simulink model "WTPG_SIM"  (R2022a)
settings: Solver=FixedStepDiscrete  StartTime=0.0  StopTime=1.08  FixedStep=0.04  RelTol=1e-3
PreLoadFcn:
  | listing = dir;
  | if (contains([listing .name], 'TCAF')) && (contains([listing .name], 'MAP'))
  |     addpath('./TCAF', './MAP');
  |     addpath( genpath('./MAP') );
  | elseif (contains([listing .name], 'WTPG.slx'))
  |     addpath('../TCAF', '../MAP');
  |     addpath( genpath('../MAP') );
  | else
  | 
  | end
  | 
  | load('BusStructureWTPG.mat');
  | load('TRN\BusStructureTRN.mat');
InitFcn:
  | listing = dir;
  | if (contains([listing .name], 'TCAF')) && (contains([listing .name], 'MAP'))
  |     addpath('./TCAF', './MAP');
  |     addpath( genpath('./MAP') );
  | elseif (contains([listing .name], 'WTPG.slx'))
  |     addpath('../TCAF', '../MAP');
  |     addpath( genpath('../MAP') );
  | else
  | 
  | end
  | 
  | load('BusStructureWTPG.mat');
  | load('TRN\BusStructureTRN.mat');
settings Model: Creator=ASCL  LastModifiedBy=ASCL
settings DataIOCC: SaveOutput=off  DSMLogging=off  SaveTime=off  ReturnWorkspaceOutputs=off
settings OptimizationCC: BlockReduction=off  DefaultParameterBehavior=Inlined  UseDivisionForNetSlopeComputation=on  GainParamInheritBuiltInType=on  UseFloatMulNetSlope=on  ExpressionFolding=off  PassReuseOutputArgsAs=Individual arguments  ZeroExternalMemoryAtStartup=off  ZeroInternalMemoryAtStartup=off  EfficientFloat2IntCast=on  LifeSpan=inf  OptimizeBlockOrder=speed  DifferentSizesBufferReuse=on  EfficientTunableParamExpr=on
settings DebuggingCC: SignalInfNanChecking=warning  ReadBeforeWriteMsg=EnableAllAsError  WriteAfterWriteMsg=EnableAllAsError  WriteAfterReadMsg=EnableAllAsError  IntegerOverflowMsg=error  ParameterTunabilityLossMsg=error  UniqueDataStoreMsg=error  AssertControl=DisableAll  NonBusSignalsTreatedAsBus=error  SFInvalidInputDataAccessInChartInitDiag=error  SFTransitionOutsideNaturalParentDiag=error  SFUnreachableExecutionPathDiag=error  SFUndirectedBroadcastEventsDiag=error  IntegerSaturationMsg=error
settings HardwareCC: ProdBitPerPointer=32  ProdBitPerSizeT=32  ProdBitPerPtrDiffT=32  ProdLargestAtomicInteger=Long  ProdLargestAtomicFloat=Double  ProdEndianess=BigEndian  ProdWordSize=32  ProdLongLongMode=on  ProdHWDeviceType=Freescale->MPC83xx
settings ModelReferenceCC: ModelReferenceNumInstancesAllowed=Single
settings SFSimCC: SimCustomHeaderCode="#include \"MAP.h\""  SimUserSources=MAP.c  SimUserLibraries=WS2_32.LIB  CompileTimeRecursionLimit=0  EnableRuntimeRecursion=off  MATLABDynamicMemAlloc=off
settings RTWCC: SystemTargetFile=ert.tlc  TemplateMakefile=ert_default_tmf  GenerateReport=on  RTWUseSimCustomCode=on  CustomHeaderCode="#include \"MAP.h\""  CustomSource=MAP.c  CustomLibrary=WS2_32.LIB  BuildConfiguration=Faster Runs  IncludeHyperlinkInReport=on  LaunchReport=on  GenerateTraceInfo=on  GenerateTraceReport=on  GenerateTraceReportSl=on  GenerateTraceReportSf=on  GenerateTraceReportEml=on
settings CodeAppCC: ForceParamTrailComments=on  IgnoreCustomStorageClasses=off  OperatorAnnotations=on  SimulinkDataObjDesc=on  SFDataObjDesc=on  MATLABFcnDesc=on  InsertBlockDesc=on  StateflowObjectComments=on  MATLABSourceComments=on  EnableCustomComments=on  InlinedPrmAccess=Macros  ReqsInCode=on
settings ERTTargetCC: TargetLangStandard=C99 (ISO)  UtilityFuncGeneration=Shared location  GenerateSampleERTMain=on  IncludeMdlTerminateFcn=off  CombineSignalStateStructs=on  SuppressErrorStatus=on  SupportAbsoluteTime=off  SupportNonFinite=off  SupportComplex=off  SupportVariableSizeSignals=on  ParenthesesLevel=Standards  CastingMode=Standards  GenerateSharedConstants=off  InlinedParameterPlacement=NonHierarchical  ERTCustomFileTemplate=example_file_process.tlc  RateTransitionBlockCode=Function  PreserveIfCondition=on  ConvertIfToSwitch=off  EnableSignedLeftShifts=off  EnableSignedRightShifts=off

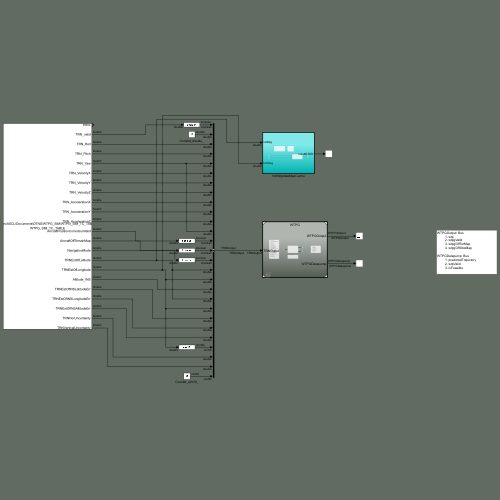
[thumbnail: Simulink's stored preview of the top-level diagram]
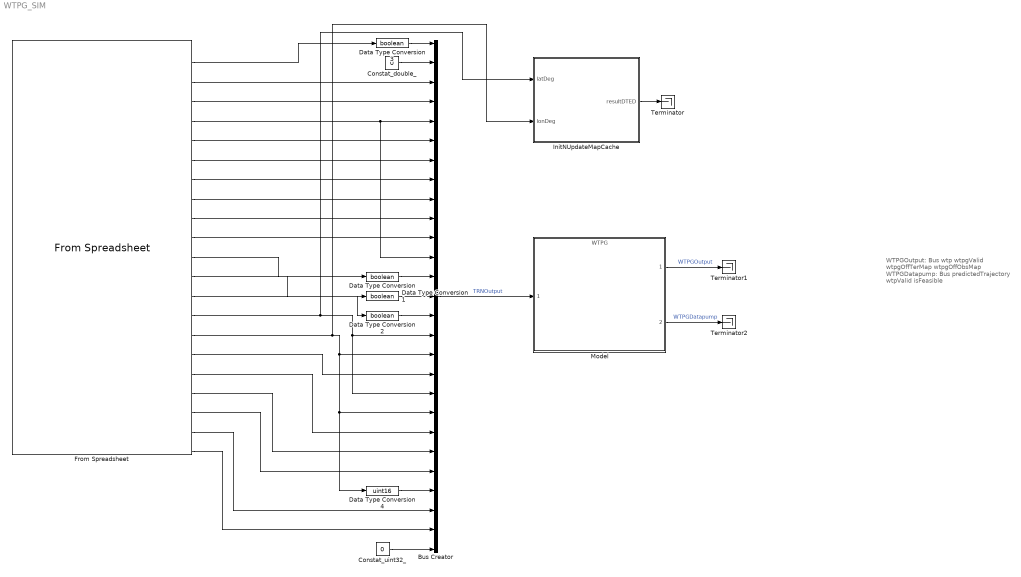
== system WTPG_SIM ==
  note: WTPGOutput: Bus
      | wtp
      | wtpgValid
      | wtpgOffTerMap
      | wtpgOffObsMap
      |
      | WTPGDatapump: Bus
      | predictedTrajectory
      | wtpValid
      | isFeasible
  Bus Creator : BusCreator  Inputs=27  OutDataTypeStr=Bus: TRNOutput  NonVirtualBus=on
      settings: InheritFromInputs=off
  Constat_double_ : Constant  Value=0  OutDataTypeStr=double
  Constat_uint32_ : Constant  Value=0  OutDataTypeStr=uint32
  Data Type Conversion{,1..3} (4 alike) : DataTypeConversion  OutDataTypeStr=boolean  RndMeth=Nearest  SaturateOnIntegerOverflow=off
  Data Type Conversion4 : DataTypeConversion  OutDataTypeStr=uint16  RndMeth=Nearest  SaturateOnIntegerOverflow=off
  From Spreadsheet : FromSpreadsheet  FileName=C:\Users\ASCL\Documents\DTNS\WTPG_SIM\WTPG_SIM_TC_TABLE.csv  SheetName=WTPG_SIM_TC_TABLE  Range=A1:V27  OutDataTypeStr=double  TreatFirstColumnAs=Data  SampleTime=0.04  OutputAfterLastPoint=Hold final value
  InitNUpdateMapCache : Subsystem  TreatAsAtomicUnit=on
  Model : ModelReference  ModelNameDialog=WTPG.slx  SimulationMode=Normal  ModelReferenceVersion=1.320
  Terminator : Terminator
  Terminator1 : Terminator
  Terminator2 : Terminator
  wires:
  Bus Creator/1 -> Model/1  "TRNOutput"
  From Spreadsheet/2 -> Data Type Conversion3/1
  From Spreadsheet/3 -> Bus Creator/3
  From Spreadsheet/4 -> Bus Creator/4
  From Spreadsheet/5 -> Bus Creator/12, Bus Creator/5
  From Spreadsheet/6 -> Bus Creator/6
  From Spreadsheet/7 -> Bus Creator/7
  From Spreadsheet/8 -> Bus Creator/8
  From Spreadsheet/9 -> Bus Creator/9
  From Spreadsheet/10 -> Bus Creator/10
  From Spreadsheet/11 -> Bus Creator/11
  From Spreadsheet/12 -> Data Type Conversion/1
  From Spreadsheet/13 -> Data Type Conversion1/1
  From Spreadsheet/14 -> Data Type Conversion2/1
  From Spreadsheet/15 -> InitNUpdateMapCache/1(latDeg), Bus Creator/16, Bus Creator/19
  From Spreadsheet/17 -> Bus Creator/18
  From Spreadsheet/19 -> Bus Creator/22
  From Spreadsheet/18 -> Bus Creator/21
  From Spreadsheet/20 -> Bus Creator/23
  Constat_uint32_/1 -> Bus Creator/27
  From Spreadsheet/22 -> Bus Creator/26
  From Spreadsheet/21 -> Bus Creator/25
  From Spreadsheet/16 -> InitNUpdateMapCache/2(lonDeg), Bus Creator/20, Data Type Conversion4/1, Bus Creator/17
  Constat_double_/1 -> Bus Creator/2
  Data Type Conversion/1 -> Bus Creator/13
  Data Type Conversion1/1 -> Bus Creator/14
  Data Type Conversion2/1 -> Bus Creator/15
  InitNUpdateMapCache/1(resultDTED) -> Terminator/1
  Model/1 -> Terminator1/1  "WTPGOutput"
  Model/2 -> Terminator2/1  "WTPGDatapump"
  Data Type Conversion3/1 -> Bus Creator/1
  Data Type Conversion4/1 -> Bus Creator/24

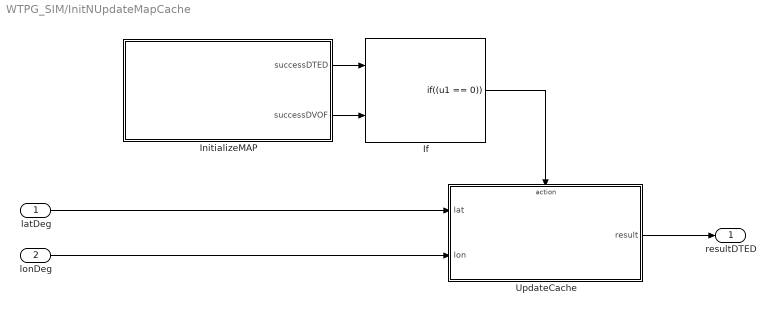
== system WTPG_SIM/InitNUpdateMapCache ==
  latDeg : Inport  OutDataTypeStr=double
  lonDeg : Inport  Port=2  OutDataTypeStr=double
  If : If  NumInputs=2  IfExpression=(u1 == 0)  ShowElse=off
  InitializeMAP : MATLAB Function  TreatAsAtomicUnit=on
  UpdateCache : Subsystem  TreatAsAtomicUnit=on
  resultDTED : Outport  VectorParamsAs1DForOutWhenUnconnected=off
  wires:
  lonDeg/1 -> UpdateCache/2(lon)
  UpdateCache/1(result) -> resultDTED/1
  InitializeMAP/1(successDTED) -> If/1
  latDeg/1 -> UpdateCache/1(lat)
  InitializeMAP/2(successDVOF) -> If/2
  If/1 -> UpdateCache/Action

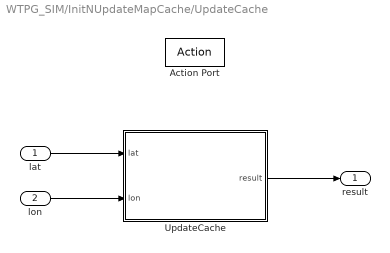
== system WTPG_SIM/InitNUpdateMapCache/UpdateCache ==
  lat : Inport
  lon : Inport  Port=2
  Action Port : ActionPort  ActionPortLabel=if((u1 == 0))
  UpdateCache : MATLAB Function  TreatAsAtomicUnit=on
  result : Outport  VectorParamsAs1DForOutWhenUnconnected=off
  wires:
  UpdateCache/1(result) -> result/1
  lat/1 -> UpdateCache/1(lat)
  lon/1 -> UpdateCache/2(lon)

== matlab function WTPG_SIM/InitNUpdateMapCache/InitializeMAP ==
  data: successDTED output; successDVOF output
function [successDTED, successDVOF] = InitializeMAP()
%InitializeMAP

% Persistent variable
persistent firstRun
if isempty(firstRun)
    firstRun = true;
end

% Initialize output
flagDTED = int32(1);
flagDVOF = int32(1);
successDTED = int32(1);
successDVOF = int32(1);

if firstRun
    % Path of DTED data
    pathDTED = 'C:\Users\ASCL\Documents\GitHub\DTNS\MAP\MAP_DB';

    % Length of DETD data path
    strLenDTED = int32(strlength(pathDTED));
    
    % Call [ InitialMap ] : 맵 폴더 위치 설정
    flagDTED = coder.ceval('InitialMap', pathDTED, strLenDTED );
    
    successDTED = flagDTED;

    if (successDTED)
        firstRun = false;
    end
else
    successDTED = int32(0);
    successDVOF = int32(0);
end

== matlab function WTPG_SIM/InitNUpdateMapCache/UpdateCache/UpdateCache ==
  data: result output; lat input; lon input
function result = UpdateCache(lat, lon)
%UpdateCache

% Persistent variables
persistent latPrev lonPrev
if isempty(latPrev)
    latPrev = 0.0;
end
if isempty(lonPrev)
    lonPrev = 0.0;
end

% Initialize output
result = int32(1);

if ( abs(lat - latPrev) > 0.05 ) || ( abs(lon - lonPrev) > 0.05)
    result = coder.ceval('UpdateCache', lat, lon);
    latPrev = lat;
    lonPrev = lon;
else
    
end
